simulink model "DX_Hand"  (R2014a)
settings: Solver=ode45  StartTime=0.0  StopTime=10.0  RelTol=1e-3
settings Model: Creator=Tonno  LastModifiedBy=Tonno
settings OptimizationCC: OptimizeModelRefInitCode=on  LifeSpan=1
settings RTWCC: SystemTargetFile=ert.tlc  GenCodeOnly=on  TemplateMakefile=ert_default_tmf  Description=Embedded Coder  ProcessScript=ert_make_rtw_hook
settings CodeAppCC: IgnoreCustomStorageClasses=off  CustomSymbolStrType=$N$R$M_Sym
settings ERTTargetCC: ParMdlRefBuildCompliant=on  CompOptLevelCompliant=on  ConcurrentExecutionCompliant=on  ERTFirstTimeCompliant=on  SupportAbsoluteTime=off  MultiInstanceERTCode=on  CodeInterfacePackaging=Reusable function  SupportNonFinite=off  SupportComplex=off  ModelStepFunctionPrototypeControlCompliant=on  CPPClassGenCompliant=on  InlinedParameterPlacement=Hierarchical  RootIOFormat=Structure reference  ERTCustomFileTemplate=example_file_process.tlc

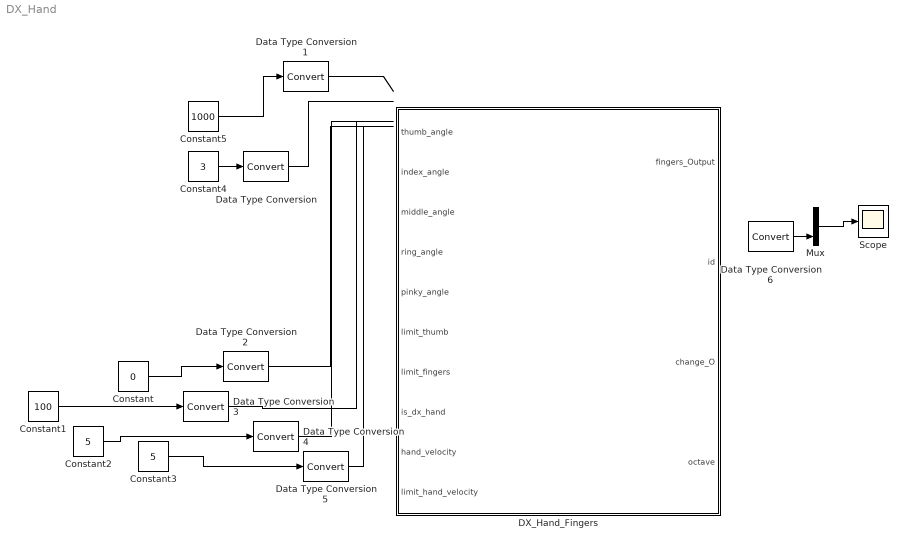
== system DX_Hand ==
  Constant : Constant  Value=0
  Constant1 : Constant  Value=100
  Constant2 : Constant  Value=5
  Constant3 : Constant  Value=5
  Constant4 : Constant  Value=3
  Constant5 : Constant  Value=1000
  "DX_Hand_Fingers " : Stateflow chart  TreatAsAtomicUnit=on
  Data Type Conversion{,1..6} (7 alike) : DataTypeConversion
  Mux : Mux  Inputs=2
  Scope : Scope
  wires:
  Constant/1 -> Data Type Conversion2/1
  Constant1/1 -> Data Type Conversion3/1
  Constant3/1 -> Data Type Conversion5/1
  Constant4/1 -> Data Type Conversion/1
  Constant5/1 -> Data Type Conversion1/1
  Data Type Conversion/1 -> ?
  Data Type Conversion1/1 -> ?
  Data Type Conversion2/1 -> ?
  Data Type Conversion3/1 -> ?
  Constant2/1 -> Data Type Conversion4/1
  Data Type Conversion4/1 -> ?
  Data Type Conversion5/1 -> ?
  ? -> Mux/1
  ? -> Data Type Conversion6/1
  Mux/1 -> Scope/1
  Data Type Conversion6/1 -> Mux/2

== stateflow chart DX_Hand/DX_Hand_Fingers  ==
  state Basic_Logic [parallel]
    during: change_O = false;
    settings: executionOrder=1
    state playing_mode
      state down
      state up
      state wait_finger
        entry: id=id+1;
        entry: fingers_Output = int32(-1);
        entry: change_O = true;
      state play_finger
        entry: id=id+1;
        entry: fingers_Output = fingers_Local;
        entry: change_O = true;
        entry: control_number= int32(0);
      wait_finger -> down [order 7] : [(hand_velocity < (-limit_hand_velocity)) && (octave>0) && (control_number<1)] / {octave = octave -int32(1);control_number= int32(1);}
      up -> wait_finger : [hand_velocity < limit_hand_velocity]
      down -> wait_finger : [hand_velocity > (-limit_hand_velocity)]
      wait_finger -> up [order 6] : [(hand_velocity > limit_hand_velocity) && (octave < 2) && (control_number<1)]/ {octave = octave + int32(1); control_number= int32(1);}
      wait_finger -> play_finger [order 1] : [thumb_angle > limit_thumb]/{fingers_Local= (int32(0) + octave*5);}
      wait_finger -> play_finger [order 2] : [index_angle > limit_fingers]/{fingers_Local= (int32(1) + octave*5);}
      wait_finger -> play_finger [order 3] : [middle_angle > limit_fingers]/{fingers_Local= (int32(2) + octave*5);}
      wait_finger -> play_finger [order 4] : [ring_angle > limit_fingers]/{fingers_Local= (int32(3) + octave*5);}
      wait_finger -> play_finger [order 5] : [pinky_angle > limit_fingers]/{fingers_Local= (int32(4) + octave*5);}
    state wait_dx_hand
      entry: id=id+1;
      entry: fingers_Output = int32(-1);
      entry: change_O = true;
      entry: control_number= int32(0);
    wait_dx_hand -> wait_finger : [is_dx_hand]
    play_finger -> wait_finger : [thumb_angle < limit_thumb && index_angle < limit_fingers && middle_angle < limit_fingers && ring_angle < limit_fingers && pinky_angle < limit_fingers]
    (default) -> wait_dx_hand : /{id= int32(0); fingers_Local = int32(-1); octave = int32(0);}
    playing_mode -> wait_dx_hand : [not(is_dx_hand)]
  data: thumb_angle input int32; index_angle input int32; middle_angle input int32; ring_angle input int32; pinky_angle input int32; limit_thumb input int32; limit_fingers input double; fingers_Local local int32; fingers_Output output int32; id output int32; is_dx_hand input boolean; change_O output boolean; hand_velocity input int32; octave output int32; limit_hand_velocity input int32; control_number local int32
